simulink model "PID_CONTROLLER"  (R2024b)
settings: Solver=VariableStepAuto  StartTime=0.0  StopTime=10.0  RelTol=1e-3
values from neighbouring files (symbols this model uses):
  Kd = 0    [matlab.mat]
  Ki = 0    [matlab.mat]
  kp = 1    [matlab.mat]
  Nf = 100    [matlab.mat]
settings Model: Creator=omari  LastModifiedBy=omari

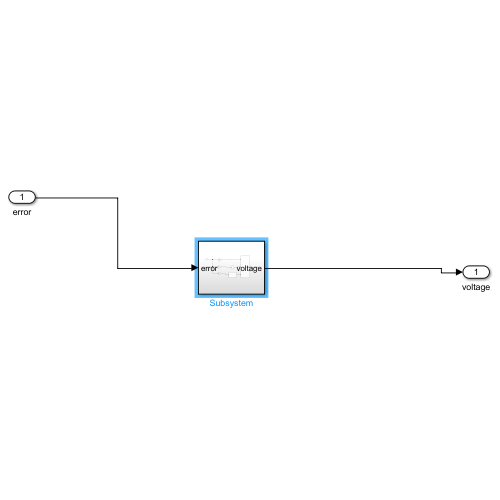
[thumbnail: Simulink's stored preview of the top-level diagram]
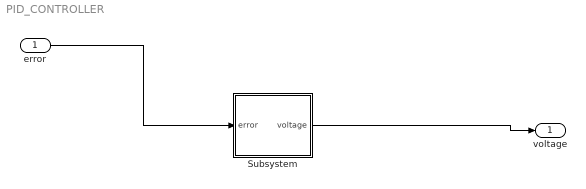
== system PID_CONTROLLER ==
  error : Inport
  Subsystem : Subsystem
  voltage : Outport
  wires:
  error/1 -> Subsystem/1(error)
  Subsystem/1(voltage) -> voltage/1

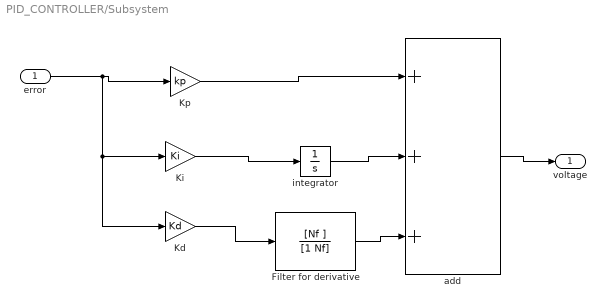
== system PID_CONTROLLER/Subsystem ==
  error : Inport
  Filter for derivative : TransferFcn  Numerator=[Nf ]  Denominator=[1 Nf]
  Kd : Gain  Gain=Kd
  Ki : Gain  Gain=Ki
  Kp : Gain  Gain=kp
  add : Sum  Inputs=+++
  integrator : Integrator
  voltage : Outport
  wires:
  error/1 -> Kd/1, Ki/1, Kp/1
  Filter for derivative/1 -> add/3
  Kd/1 -> Filter for derivative/1
  Kp/1 -> add/1
  integrator/1 -> add/2
  Ki/1 -> integrator/1
  add/1 -> voltage/1
